simulink model "Sensing"  (R2024b)
settings: Solver=ode1  StartTime=0.0  StopTime=10.0  FixedStep=0.5e-3  RelTol=1e-3
settings Model: DataDictionary=Sensing_dd.sldd  EnableAccessToBaseWorkspace=off  Creator=wai484  LastModifiedBy=wai484
settings DataIOCC: SaveOutput=off  SignalLogging=off  DSMLogging=off  SaveTime=off  ReturnWorkspaceOutputs=off
settings OptimizationCC: UseDivisionForNetSlopeComputation=UseDivisionForReciprocalsOfIntegersOnly  StateBitsets=on  DataBitsets=on  EfficientFloat2IntCast=on
settings DebuggingCC: SignalInfNanChecking=error  ReadBeforeWriteMsg=EnableAllAsError  WriteAfterWriteMsg=EnableAllAsError  WriteAfterReadMsg=EnableAllAsError  AlgebraicLoopMsg=error  ArtificialAlgebraicLoopMsg=error  SaveWithDisabledLinksMsg=error  SaveWithParameterizedLinksMsg=error  BlockPriorityViolationMsg=error  TimeAdjustmentMsg=warning  InheritedTsInSrcMsg=error  SingleTaskRateTransMsg=error  TasksWithSamePriorityMsg=error  SigSpecEnsureSampleTimeMsg=error  CheckMatrixSingularityMsg=error  IntegerOverflowMsg=error  ParameterUnderflowMsg=error  ParameterPrecisionLossMsg=error  ParameterTunabilityLossMsg=error  FixptConstUnderflowMsg=error  FixptConstOverflowMsg=error  FixptConstPrecisionLossMsg=error  UnderSpecifiedDataTypeMsg=error  UnnecessaryDatatypeConvMsg=warning  VectorMatrixConversionMsg=error  UnconnectedInputMsg=error  UnconnectedOutputMsg=error  UnconnectedLineMsg=error  SFcnCompatibilityMsg=error  UniqueDataStoreMsg=error  BusObjectLabelMismatch=error  RootOutportRequireBusObject=error  AssertControl=DisableAll  ModelReferenceVersionMismatchMessage=error  ModelReferenceIOMismatchMessage=error  UnknownTsInhSupMsg=error  ModelReferenceDataLoggingMessage=error  StateNameClashWarn=warning  OperatingPointInterfaceChecksumMismatchMsg=error  StrictBusMsg=ErrorOnBusTreatedAsVector  NonBusSignalsTreatedAsBus=error  SFUnusedDataAndEventsDiag=error  SFInvalidInputDataAccessInChartInitDiag=error  SFTransitionOutsideNaturalParentDiag=error  SFUnreachableExecutionPathDiag=error  SFUndirectedBroadcastEventsDiag=error  SFTransitionActionBeforeConditionDiag=error  SFTemporalDelaySmallerThanSampleTimeDiag=error  SFSelfTransitionDiag=error  SFExecutionAtInitializationDiag=error  IntegerSaturationMsg=error  UnderSpecifiedDimensionMsg=error  VariantConditionMismatch=error  InheritVATfromSVC=error  VariantConfigNotUsedByTopModel=error
settings ModelReferenceCC: EnableParallelModelReferenceBuilds=on
settings SFSimCC: CompileTimeRecursionLimit=0  EnableRuntimeRecursion=off  MATLABDynamicMemAlloc=off
settings RTWCC: BuildConfiguration=Faster Runs
settings CodeAppCC: ForceParamTrailComments=on  StateflowObjectComments=on  MATLABSourceComments=on
settings GRTTargetCC: UtilityFuncGeneration=Shared location  MatFileLogging=off  SupportNonFinite=off  GenerateSharedConstants=off  OptimizeReductions=on

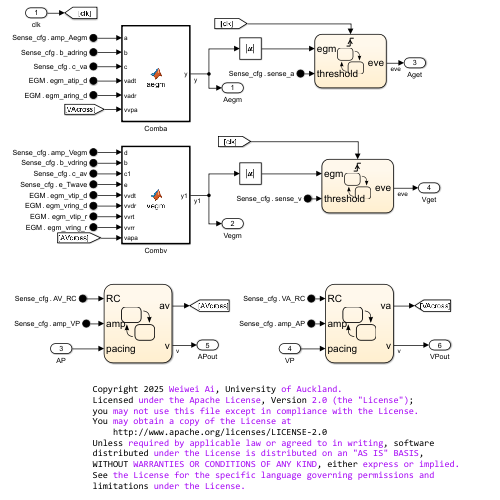
[thumbnail: Simulink's stored preview of the top-level diagram]
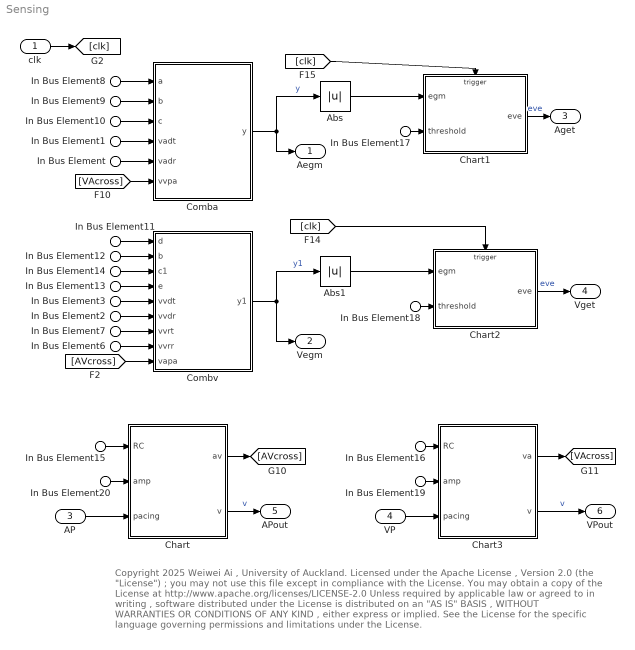
== system Sensing ==
  note: Copyright 2025 Weiwei Ai , University of Auckland.
      | Licensed under the Apache License , Version 2.0 (the "License") ;
      | you may not use this file except in compliance with the License.
      | You may obtain a copy of the License at
      | http://www.apache.org/licenses/LICENSE-2.0
      | Unless required by applicable law or agreed to in writing , software
      | distributed under the License is distributed on an "AS IS" BASIS ,
      | WITHOUT WARRANTIES OR CONDITIONS OF ANY KIND , either express or implied.
      | See the License for the specific language governing permissions and
      | limitations under the License.
  clk : Inport  OutDataTypeStr=double  PortDimensions=1
  In Bus Element : Inport  Port=2  PortName=EGM  Element=aring_d
  In Bus Element1 : Inport  Port=2  PortName=EGM  Element=atip_d
  In Bus Element2 : Inport  Port=2  PortName=EGM  Element=vring_d
  In Bus Element3 : Inport  Port=2  PortName=EGM  Element=vtip_d
  In Bus Element6 : Inport  Port=2  PortName=EGM  Element=vring_r
  In Bus Element7 : Inport  Port=2  PortName=EGM  Element=vtip_r
  AP : Inport  Port=3  OutDataTypeStr=double  PortDimensions=1
  VP : Inport  Port=4  OutDataTypeStr=double  PortDimensions=1
  In Bus Element8 : Inport  Port=5  PortName=Sense_cfg  Element=amp_Aegm
  In Bus Element9 : Inport  Port=5  PortName=Sense_cfg  Element=b_adring
  In Bus Element10 : Inport  Port=5  PortName=Sense_cfg  Element=c_va
  In Bus Element11 : Inport  Port=5  PortName=Sense_cfg  Element=amp_Vegm
  In Bus Element12 : Inport  Port=5  PortName=Sense_cfg  Element=b_vdring
  In Bus Element13 : Inport  Port=5  PortName=Sense_cfg  Element=e_Twave
  In Bus Element14 : Inport  Port=5  PortName=Sense_cfg  Element=c_av
  In Bus Element15 : Inport  Port=5  PortName=Sense_cfg  Element=AV_RC
  In Bus Element16 : Inport  Port=5  PortName=Sense_cfg  Element=VA_RC
  In Bus Element17 : Inport  Port=5  PortName=Sense_cfg  Element=sense_a
  In Bus Element18 : Inport  Port=5  PortName=Sense_cfg  Element=sense_v
  In Bus Element19 : Inport  Port=5  PortName=Sense_cfg  Element=amp_AP
  In Bus Element20 : Inport  Port=5  PortName=Sense_cfg  Element=amp_VP
  Abs : Abs  SaturateOnIntegerOverflow=off
  Abs1 : Abs  SaturateOnIntegerOverflow=off
  Chart : Stateflow chart  TreatAsAtomicUnit=on
  Chart1 : Stateflow chart  TreatAsAtomicUnit=on
  Chart2 : Stateflow chart  TreatAsAtomicUnit=on
  Chart3 : Stateflow chart  TreatAsAtomicUnit=on
  Comba : MATLAB Function  TreatAsAtomicUnit=on
  Combv : MATLAB Function  TreatAsAtomicUnit=on
  Aegm : Outport  OutDataTypeStr=double  PortDimensions=1  SampleTime=[0,1]
  Vegm : Outport  Port=2  OutDataTypeStr=double  PortDimensions=1  SampleTime=[0,1]
  Aget : Outport  Port=3  OutDataTypeStr=double  PortDimensions=1
  Vget : Outport  Port=4  OutDataTypeStr=double  PortDimensions=1
  APout : Outport  Port=5  OutDataTypeStr=double  PortDimensions=1  SampleTime=[0,1]
  VPout : Outport  Port=6  OutDataTypeStr=double  PortDimensions=1  SampleTime=[0,1]
  wires:
  Comba/1(y) -> Abs/1, Aegm/1  "y"
  AP/1 -> Chart/3(pacing)
  VP/1 -> Chart3/3(pacing)
  In Bus Element1/1 -> Comba/4(vadt)
  In Bus Element/1 -> Comba/5(vadr)
  Combv/1(y1) -> Vegm/1, Abs1/1  "y1"
  [AVcross] -> Combv/9(vapa)
  [VAcross] -> Comba/6(vvpa)
  Chart/2(v) -> APout/1  "v"
  Chart3/1(va) -> [VAcross]
  Chart3/2(v) -> VPout/1  "v"
  Chart1/1(eve) -> Aget/1  "eve"
  Abs/1 -> Chart1/1(egm)
  clk/1 -> [clk]
  [clk] -> Chart1/Trigger
  Chart2/1(eve) -> Vget/1  "eve"
  Abs1/1 -> Chart2/1(egm)
  [clk] -> Chart2/Trigger
  In Bus Element8/1 -> Comba/1(a)
  In Bus Element9/1 -> Comba/2(b)
  In Bus Element10/1 -> Comba/3(c)
  In Bus Element11/1 -> Combv/1(d)
  In Bus Element12/1 -> Combv/2(b)
  In Bus Element13/1 -> Combv/4(e)
  In Bus Element14/1 -> Combv/3(c1)
  In Bus Element3/1 -> Combv/5(vvdt)
  In Bus Element2/1 -> Combv/6(vvdr)
  In Bus Element7/1 -> Combv/7(vvrt)
  In Bus Element6/1 -> Combv/8(vvrr)
  Chart/1(av) -> [AVcross]
  In Bus Element15/1 -> Chart/1(RC)
  In Bus Element16/1 -> Chart3/1(RC)
  In Bus Element20/1 -> Chart/2(amp)
  In Bus Element19/1 -> Chart3/2(amp)
  In Bus Element17/1 -> Chart1/2(threshold)
  In Bus Element18/1 -> Chart2/2(threshold)

== matlab function Sensing/Combv ==
  data: d input; y1 output; b input; c1 input; e input; vvdt input; vvdr input; vvrt input; vvrr input; vapa input
function y1 = vegm(d,b,c1,e,vvdt,vvdr,vvrt,vvrr,vapa)
%#codegen
%VEGM Combine possible signals sensed by the ventricular lead.
%   d, b, c1, e are used to determine which signals are present to the device.
%
%   Inputs:
%       d - Weight for the amplitude of Aegm
%       b - Weight for the amplitude of the signal sensed by the ring
%       electrodes. When b=0, the output is unipolar.          
%       c1 - Scale the atrial pacing artifact (i.e.,AV crosstalk)
%       vvdt - Signal sensed by the tip electrodes (depolarisation).
%       vvdr - Signal sensed by the ring electrodes (depolarisation).
%       vvrt - Signal sensed by the tip electrodes (repolarisation).
%       vvrr - Signal sensed by the ring electrodes (repolarisation).
%       vapa - Atrial pacing artifact/afterpotentials (i.e.,AV crosstalk)

%   Outputs:
%       y - Signals sensed by the ventricular lead
y1 = d*(vvdt-b*vvdr+e*(vvrt-b*vvrr)+c1*vapa);

== stateflow chart Sensing/Chart1 ==
  settings: executeAtInitialization=1
  state Ini
  Ini -> Ini [order 1] : clk[egm>=threshold]/{eve=1;}
  (default) -> Ini
  Ini -> Ini [order 2] : clk[egm<threshold]/{eve=0;}
  data: egm input; threshold input; eve output
  events: clk input RISING_EDGE_EVENT

== stateflow chart Sensing/Chart3 ==
  settings: executeAtInitialization=1
  state S
    state After_potential [parallel]
      settings: executionOrder=1
      state Timer
        du:
        t=temporalCount(msec);
        va=exp(-t)/RC;
      state Ini
      state waith
      waith -> S.After_potential.Timer : [pacing==0]
      (default) -> S.After_potential.Ini : /{t=0;va=0;}
      S.After_potential.Ini -> waith : [pacing>=1]
      S.After_potential.Timer -> waith : [pacing>=1]/{t=0;va=0;}
    state Pulse [parallel]
      settings: executionOrder=2
      state Ini
      state Timer
        du:
        t1=temporalCount(msec);
        v=amp;
      state waitl
      S.Pulse.Ini -> S.Pulse.Timer : [pacing>=1]
      (default) -> S.Pulse.Ini : /{t1=0;v=0;}
      waitl -> S.Pulse.Ini : [pacing==0]
      S.Pulse.Timer -> waitl : [after(3,msec)]/{v=0;}
  (default) -> S
  data: va output; t local; RC input; v output; t1 local; amp input; pacing input

== stateflow chart Sensing/Chart ==
  settings: executeAtInitialization=1
  state S
    state After_potential [parallel]
      settings: executionOrder=1
      state Timer
        du:
        t=temporalCount(msec);
        av=exp(-t)/RC;
      state Ini
      state waith
      waith -> S.After_potential.Timer : [pacing==0]
      (default) -> S.After_potential.Ini : /{t=0;av=0;}
      S.After_potential.Ini -> waith : [pacing>=1]
      S.After_potential.Timer -> waith : [pacing>=1]/{t=0;av=0;}
    state Pulse [parallel]
      settings: executionOrder=2
      state Ini
      state Timer
        du:
        t1=temporalCount(msec);
        v=amp;
      state waitl
      S.Pulse.Ini -> S.Pulse.Timer : [pacing>=1]
      (default) -> S.Pulse.Ini : /{t1=0;v=0;}
      waitl -> S.Pulse.Ini : [pacing==0]
      S.Pulse.Timer -> waitl : [after(3,msec)]/{v=0;}
  (default) -> S
  data: av output; t local; RC input; v output; t1 local; amp input; pacing input

== stateflow chart Sensing/Chart2 ==
  settings: executeAtInitialization=1
  state Ini
  Ini -> Ini [order 1] : clk[egm>=threshold]/{eve=1;}
  (default) -> Ini
  Ini -> Ini [order 2] : clk[egm<threshold]/{eve=0;}
  data: egm input; threshold input; eve output
  events: clk input RISING_EDGE_EVENT

== matlab function Sensing/Comba ==
  data: a input; y output; b input; c input; vadt input; vadr input; vvpa input
function y = aegm(a,b,c,vadt,vadr,vvpa)
%#codegen
%AEGM Combine possible signals sensed by the atrial lead.
%   a, b, c are used to determine which signals are present to the device.
%
%   Inputs:
%       a - Weight for the amplitude of Aegm
%       b - Weight for the amplitude of the signal sensed by the ring
%       electrodes. When b=0, the output is unipolar.          
%       c - Scale the ventricular pacing artifact (i.e.,VA crosstalk)
%       vadt - Signal sensed by the tip electrodes (depolarisation).
%       vadr - Signal sensed by the ring electrodes (depolarisation).
%       vvpa - Ventricular pacing artifact/afterpotentials (i.e.,VA crosstalk)

%   Outputs:
%       y - Signals sensed by the atrial lead


y = a*(vadt-b*vadr+c*vvpa);
